simulink model "Rx_BPSK_delta_RTL_SDR_light"  (Simulink 7.4)
settings: Solver=ode45  StartTime=0.0  StopTime=inf  RelTol=1e-3
undefined symbols (not defined in the file): get
libraries: dspbuff3 x6, commutil2 x2, dspmlti4 x2, dspsnks4 x2, dsparch4 x1, commsink2 x1, simulink x1, commfilt2 x1, commtimrec2 x1, rtlsdr x1
settings Model: Creator=wnieves  LastModifiedBy=Bscheers
settings OptimizationCC: InitFltsAndDblsToZero=on

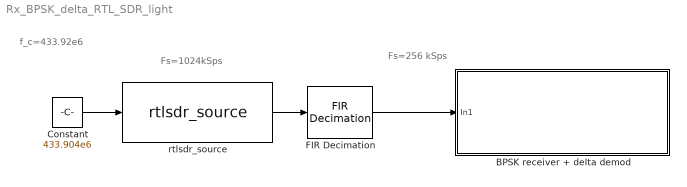
== system Rx_BPSK_delta_RTL_SDR_light ==
  note: f_c=433.92e6
  note: Fs=256 kSps
  note: Fs=1024kSps
  BPSK receiver + delta demod : Subsystem
      mask Display: fprintf('Receiver')
  Constant : Constant  Value=433.904e6  OutDataType=fixdt(1, 16)  OutScaling=2^0
  FIR Decimation : dspmlti4/FIR Decimation  DialogController=dspdialog.FIRDecimation  DialogControllerArgs=DataTag5  h=fir1(20,0.125)  D=4  filtStruct=Direct form  framing=Maintain input frame rate  outputBufInitCond=0  roundingMode=Floor  overflowMode=off  FilterSource=Specify via dialog  FilterObject=Hm_firdecim
  rtlsdr_source : rtlsdr/rtlsdr_source  rtlsdr_device_index=0  rtlsdr_query=off  rtlsdr_samplerate=1024e3  rtlsdr_frame_length=2048*8  rtlsdr_frame_type=Frame  rtlsdr_frequency=100.6e6  rtlsdr_frequency_tune=on  rtlsdr_gain=19.1  rtlsdr_gain_tune=off  rtlsdr_agc_on=on  rtlsdr_restore_block=off
  wires:
  rtlsdr_source/1 -> FIR Decimation/1
  Constant/1 -> rtlsdr_source/1
  FIR Decimation/1 -> BPSK receiver + delta demod/1(In1)

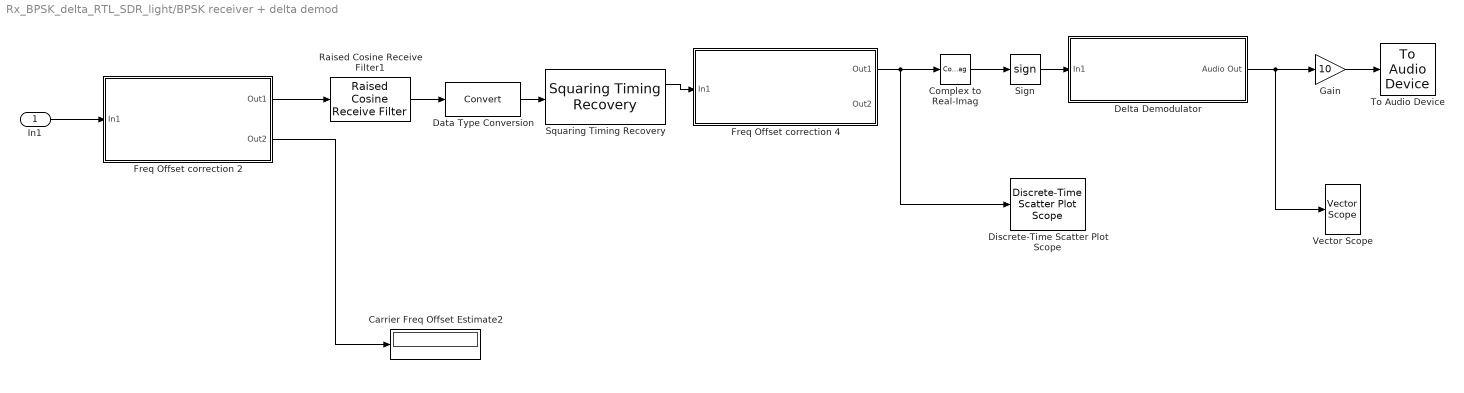
== system Rx_BPSK_delta_RTL_SDR_light/BPSK receiver + delta demod ==
  In1 : Inport  OutDataType=fixdt(1, 16)  OutScaling=2^0
  Carrier Freq Offset Estimate2 : Display
  Complex to Real-Imag : ComplexToRealImag  Output=Real
  Data Type Conversion : DataTypeConversion  OutDataType=fixdt(1, 16)  OutScaling=2^0
  Delta Demodulator : Subsystem
  Discrete-Time Scatter Plot Scope : commsink2/Discrete-Time Scatter Plot Scope  Tag=ScatterPlot  SystemSampleTime=-1  sampPerSymb=1  offsetEye=0  numTraces=40  numNewFrames=10  LineMarkers=.  LineColors=b  fading=on  render=on  AxisGrid=on  xMin=-1.60978085285153  xMax=1.62663894428818  yMin=-1.63581285423745  yMax=1.60060694290226  inphaseLabel=In-phase Amplitude  quadratureLabel=Quadrature Amplitude  openScopeAtSimStart=on  FrameNumber=off  FigPos=get(0,'defaultfigureposition');  figTitle=Scatter Plot  numLinesMax=8  block_type_=scatter
  Freq Offset correction 2 : Subsystem
      mask Display: fprintf('Coarse Freq Offset Estimater \n Delay-and-Multiply')
  Freq Offset correction 4 : Subsystem
      mask Display: fprintf('Costas Loop');
  Gain : Gain  Gain=10  ParameterDataType=fixdt(1, 16)  ParameterScaling=2^0  OutDataType=fixdt(1, 16)  OutScaling=2^0
  Raised Cosine Receive Filter1 : commfilt2/Raised Cosine Receive Filter  DialogController=dspDDGCreate  DialogControllerArgs=DataTag2  SystemSampleTime=-1  filtType=Square root  N=16  D=8  R=0.35  sampMode=Mute  saveAsFlag=0  framing=Maintain input frame rate  rateMode=None  downFactor=8  downOffset=0  checkGain=Normalized  filterGain=1  checkCoeff=off  variableName=rcRxFilt1  launchFVT=off  roundingMode=Floor  overflowMode=off
  Sign : Signum
  Squaring Timing Recovery : commtimrec2/Squaring Timing Recovery  SystemSampleTime=-1  numSymb=256  sampPerSymb=16
  To Audio Device : dspsnks4/To Audio Device  DialogController=dspDDGCreate  DialogControllerArgs=DataTag3  deviceName=Default  inheritSampleRate=off  sampleRate=16000  deviceDatatype=Determine from input data type  autoBufferSize=on  bufferSize=4096  queueDuration=1.0
  Vector Scope : dspsnks4/Vector Scope  DialogController=dspdialog.VectorScope  DialogControllerArgs=DataTag4  ScopeProperties=on  Domain=Time  HorizSpan=1  DisplayProperties=off  AxisGrid=on  Memory=off  FrameNumber=on  AxisLegend=off  AxisZoom=off  OpenScopeAtSimStart=on  OpenScopeImmediately=off  FigPos=get(0,'defaultfigureposition')  AxisProperties=off  XUnits=Hertz  XRange=[0...Fs/2]  InheritXIncr=on  XIncr=1  XLabel=Time  XLimit=Auto  XMin=0  XMax=1  XStart=0  YUnits=dB  YLabel=Amplitude  LineProperties=off  XAxisParamsVer=6.9
      settings: YMin=-10  YMax=10
  wires:
  Gain/1 -> To Audio Device/1
  Delta Demodulator/1(Audio Out) -> Gain/1, Vector Scope/1
  Complex to Real-Imag/1 -> Sign/1
  Sign/1 -> Delta Demodulator/1(In1)
  In1/1 -> Freq Offset correction 2/1(In1)
  Data Type Conversion/1 -> Squaring Timing Recovery/1
  Freq Offset correction 4/1(Out1) -> Complex to Real-Imag/1, Discrete-Time Scatter Plot Scope/1
  Squaring Timing Recovery/1 -> Freq Offset correction 4/1(In1)
  Freq Offset correction 2/2(Out2) -> Carrier Freq Offset Estimate2/1
  Raised Cosine Receive Filter1/1 -> Data Type Conversion/1
  Freq Offset correction 2/1(Out1) -> Raised Cosine Receive Filter1/1

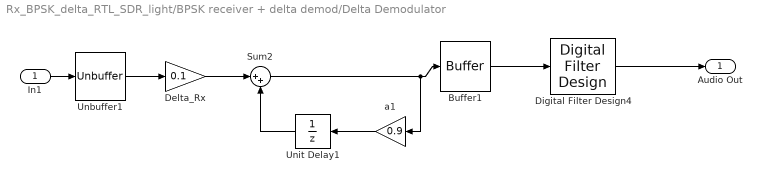
== system Rx_BPSK_delta_RTL_SDR_light/BPSK receiver + delta demod/Delta Demodulator ==
  In1 : Inport
  Buffer1 : dspbuff3/Buffer  N=256  V=0  ic=0
  Delta_Rx : Gain  Gain=0.1  ParameterDataType=sfix(16)  ParameterScaling=2^0  OutDataType=sfix(16)  OutScaling=2^0
  Digital Filter Design4 : dsparch4/Digital Filter Design  SystemSampleTime=-1  mwdsp_browser_bugfix_var=off
  Sum2 : Sum  Inputs=|++  OutDataType=sfix(16)  OutScaling=2^0
  Unbuffer1 : dspbuff3/Unbuffer  ic=0
  Unit Delay1 : UnitDelay  SampleTime=-1
  a1 : Gain  Gain=0.9  ParameterDataType=sfix(16)  ParameterScaling=2^0  OutDataType=sfix(16)  OutScaling=2^0
  Audio Out : Outport
  wires:
  Delta_Rx/1 -> Sum2/1
  a1/1 -> Unit Delay1/1
  Unit Delay1/1 -> Sum2/2
  Sum2/1 -> a1/1, Buffer1/1
  Unbuffer1/1 -> Delta_Rx/1
  In1/1 -> Unbuffer1/1
  Buffer1/1 -> Digital Filter Design4/1
  Digital Filter Design4/1 -> Audio Out/1

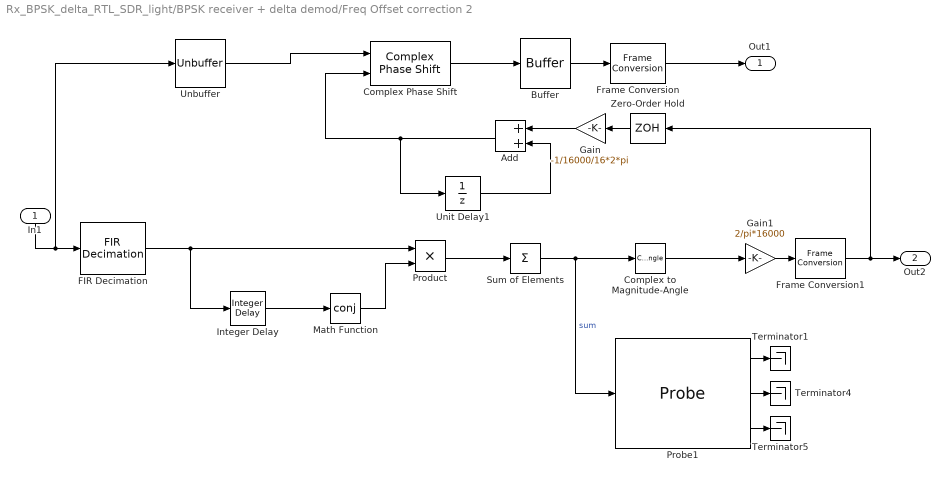
== system Rx_BPSK_delta_RTL_SDR_light/BPSK receiver + delta demod/Freq Offset correction 2 ==
  In1 : Inport
  Add : Sum  OutDataType=fixdt(1, 16)  OutScaling=2^-10
  Buffer : dspbuff3/Buffer  N=4096  V=0  ic=0
  Complex Phase Shift : commutil2/Complex Phase Shift  SystemSampleTime=-1
  Complex to Magnitude-Angle : ComplexToMagnitudeAngle  Output=Angle
  FIR Decimation : dspmlti4/FIR Decimation  DialogController=dspdialog.FIRDecimation  DialogControllerArgs=DataTag1  h=fir1(35,0.125)  D=4  filtStruct=Direct form  framing=Maintain input frame rate  outputBufInitCond=0  roundingMode=Floor  overflowMode=off  FilterSource=Specify via dialog  FilterObject=Hm_firdecim
  Frame Conversion : FrameConversion
  Frame Conversion1 : FrameConversion  OutFrame=Sample-based
  Gain : Gain  Gain=-1/16000/16*2*pi  ParameterDataType=fixdt(1, 16)  ParameterScaling=2^0  OutDataType=fixdt(1, 16)  OutScaling=2^0
  Gain1 : Gain  Gain=2/pi*16000  ParameterDataType=fixdt(1, 16)  ParameterScaling=2^0  OutDataType=fixdt(1, 16)  OutScaling=2^0
  Integer Delay : simulink/Discrete/Integer Delay  vinit=0.0  samptime=-1  NumDelays=1
  Math Function : Math  Operator=conj  OutDataType=fixdt(1, 16)  OutScaling=2^0  SaturateOnIntegerOverflow=on
  Probe1 : Probe  ProbeComplexSignal=off  ProbeFramedSignal=on
  Product : Product  OutDataType=fixdt(1, 16)  OutScaling=2^0  RndMeth=Zero
  Sum of Elements : Sum  Inputs=+  OutDataType=fixdt(1, 16)  OutScaling=2^-10
  Terminator1 : Terminator
  Terminator4 : Terminator
  Terminator5 : Terminator
  Unbuffer : dspbuff3/Unbuffer  ic=0
  Unit Delay1 : UnitDelay  SampleTime=-1
  Zero-Order Hold : ZeroOrderHold  SampleTime=1/16000/16
  Out1 : Outport
  Out2 : Outport  Port=2
  wires:
  Frame Conversion1/1 -> Out2/1, Zero-Order Hold/1
  Probe1/3 -> Terminator5/1
  Probe1/2 -> Terminator4/1
  Probe1/1 -> Terminator1/1
  FIR Decimation/1 -> Integer Delay/1, Product/1
  Gain1/1 -> Frame Conversion1/1
  In1/1 -> FIR Decimation/1, Unbuffer/1
  Complex to Magnitude-Angle/1 -> Gain1/1
  Sum of Elements/1 -> Probe1/1, Complex to Magnitude-Angle/1  "sum"
  Product/1 -> Sum of Elements/1
  Math Function/1 -> Product/2
  Integer Delay/1 -> Math Function/1
  Unbuffer/1 -> Complex Phase Shift/1
  Complex Phase Shift/1 -> Buffer/1
  Buffer/1 -> Frame Conversion/1
  Gain/1 -> Add/1
  Add/1 -> Unit Delay1/1, Complex Phase Shift/2
  Unit Delay1/1 -> Add/2
  Zero-Order Hold/1 -> Gain/1
  Frame Conversion/1 -> Out1/1

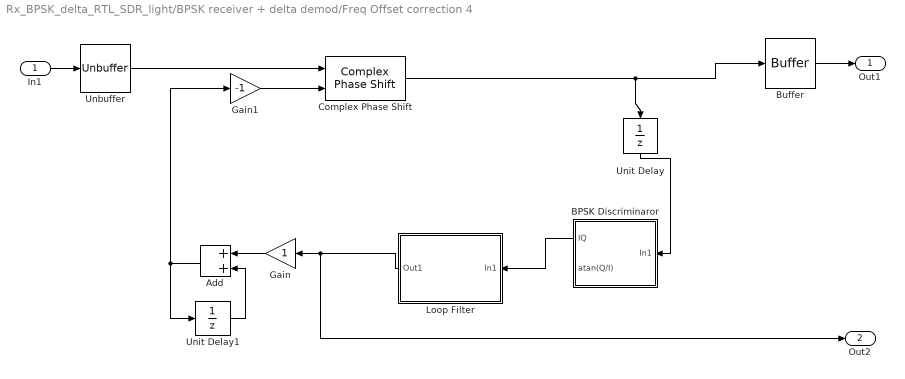
== system Rx_BPSK_delta_RTL_SDR_light/BPSK receiver + delta demod/Freq Offset correction 4 ==
  In1 : Inport
  Add : Sum  OutDataType=fixdt(1, 16)  OutScaling=2^-10
  BPSK Discriminaror : Subsystem
  Buffer : dspbuff3/Buffer  N=256  V=0  ic=0
  Complex Phase Shift : commutil2/Complex Phase Shift  SystemSampleTime=-1
  Gain : Gain  ParameterDataType=fixdt(1, 16)  ParameterScaling=2^0  OutDataType=fixdt(1, 16)  OutScaling=2^0
  Gain1 : Gain  Gain=-1  ParameterDataType=fixdt(1, 16)  ParameterScaling=2^0  OutDataType=fixdt(1, 16)  OutScaling=2^0
  Loop Filter : Subsystem
  Unbuffer : dspbuff3/Unbuffer  ic=0
  Unit Delay : UnitDelay  SampleTime=-1
  Unit Delay1 : UnitDelay  SampleTime=-1
  Out1 : Outport
  Out2 : Outport  Port=2
  wires:
  Gain1/1 -> Complex Phase Shift/2
  Gain/1 -> Add/1
  Unit Delay1/1 -> Add/2
  Add/1 -> Gain1/1, Unit Delay1/1
  Buffer/1 -> Out1/1
  In1/1 -> Unbuffer/1
  Unbuffer/1 -> Complex Phase Shift/1
  Complex Phase Shift/1 -> Buffer/1, Unit Delay/1
  Unit Delay/1 -> BPSK Discriminaror/1(In1)
  Loop Filter/1(Out1) -> Out2/1, Gain/1
  BPSK Discriminaror/1(IQ) -> Loop Filter/1(In1)

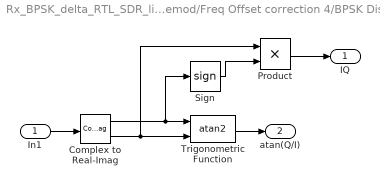
== system Rx_BPSK_delta_RTL_SDR_light/BPSK receiver + delta demod/Freq Offset correction 4/BPSK Discriminaror ==
  In1 : Inport
  Complex to Real-Imag : ComplexToRealImag
  Product : Product  OutDataType=fixdt(1, 16)  OutScaling=2^0  RndMeth=Zero
  Sign : Signum
  Trigonometric Function : Trigonometry  Operator=atan2
  IQ : Outport
  atan(Q/I) : Outport  Port=2
  wires:
  Sign/1 -> Product/2
  Product/1 -> IQ/1
  In1/1 -> Complex to Real-Imag/1
  Complex to Real-Imag/1 -> Sign/1, Trigonometric Function/1
  Complex to Real-Imag/2 -> Product/1, Trigonometric Function/2
  Trigonometric Function/1 -> atan(Q/I)/1

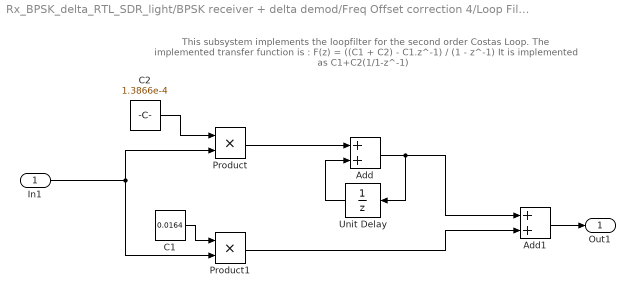
== system Rx_BPSK_delta_RTL_SDR_light/BPSK receiver + delta demod/Freq Offset correction 4/Loop Filter ==
  note: This subsystem implements the loopfilter for the second order Costas Loop. The implemented
      | transfer function is : F(z) = ((C1 + C2) - C1.z^-1) / (1 - z^-1)
      |
      | It is implemented as C1+C2(1/1-z^-1)
  In1 : Inport  OutDataType=fixdt(1, 16)  OutScaling=2^0
  Add : Sum  OutDataType=fixdt(1, 16)  OutScaling=2^-10
  Add1 : Sum  OutDataType=fixdt(1, 16)  OutScaling=2^-10
  C1 : Constant  Value=0.0164  OutDataTypeMode=single  OutDataType=fixdt(1, 16)  OutScaling=2^0  OutDataTypeStr=single
  C2 : Constant  Value=1.3866e-4  OutDataTypeMode=single  OutDataType=fixdt(1, 16)  OutScaling=2^0  OutDataTypeStr=single
  Product : Product  OutDataType=fixdt(1, 16)  OutScaling=2^0  RndMeth=Zero
  Product1 : Product  OutDataType=fixdt(1, 16)  OutScaling=2^0  RndMeth=Zero
  Unit Delay : UnitDelay  X0=0.1  SampleTime=-1
  Out1 : Outport  OutDataType=fixdt(1, 16)  OutScaling=2^0
  wires:
  C2/1 -> Product/1
  In1/1 -> Product/2, Product1/2
  Product/1 -> Add/1
  Product1/1 -> Add1/2
  Add/1 -> Add1/1, Unit Delay/1
  Unit Delay/1 -> Add/2
  Add1/1 -> Out1/1
  C1/1 -> Product1/1
